simulink model "Project0x2DMPPTControl (2)"  (R2024a)
settings: Solver=FixedStepDiscrete  StartTime=0.0  StopTime=inf  FixedStep=10e-6  RelTol=1e-3
undefined symbols (not defined in the file): Ion, Lithium
libraries: spsSeriesRLCBranchLib x9, spsIGBTDiodeLib x3, slpidlib x2, spsPWMGeneratorDCDCLib x2, spsBatteryLib x1, spsCurrentMeasurementLib x1, spsDiodeLib x1, spsPVArrayLib x1, spsVoltageMeasurementLib x1, spspowerguiLib x1
settings Model: Creator=SHADMAN  LastModifiedBy=deept

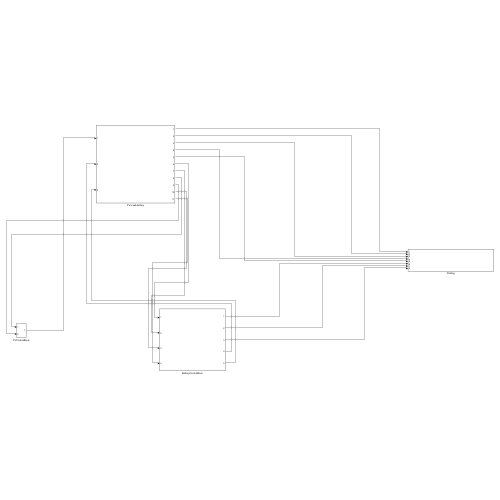
[thumbnail: Simulink's stored preview of the top-level diagram]
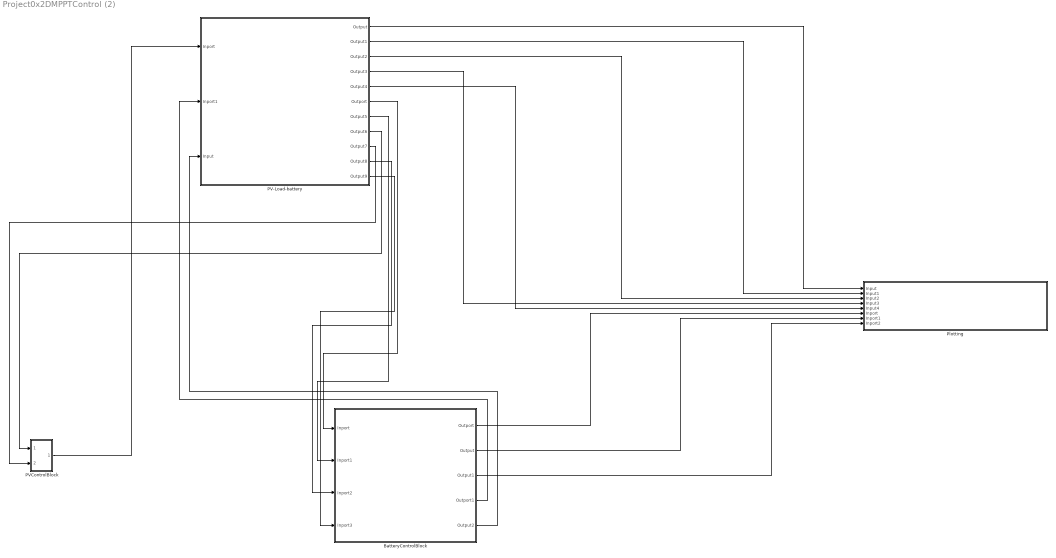
== system Project0x2DMPPTControl (2) ==
  BatteryControlBlock : Subsystem
  PV-Load-battery : Subsystem
  PVControlBlock : Subsystem
  Plotting : Subsystem
  wires:
  PV-Load-battery/1(Output) -> Plotting/1(Input)
  PV-Load-battery/2(Output1) -> Plotting/2(Input1)
  PV-Load-battery/4(Output3) -> Plotting/4(Input3)
  PV-Load-battery/5(Output4) -> Plotting/5(Input4)
  PV-Load-battery/3(Output2) -> Plotting/3(Input2)
  BatteryControlBlock/1(Outport) -> Plotting/6(Inport)
  BatteryControlBlock/2(Output) -> Plotting/7(Inport1)
  BatteryControlBlock/3(Output1) -> Plotting/8(Inport2)
  PVControlBlock/1(Outport) -> PV-Load-battery/1(Inport)
  PV-Load-battery/6(Outport) -> BatteryControlBlock/1(Inport)
  PV-Load-battery/7(Output5) -> BatteryControlBlock/2(Inport1)
  PV-Load-battery/8(Output6) -> PVControlBlock/1(Inport)
  PV-Load-battery/9(Output7) -> PVControlBlock/2(Input)
  PV-Load-battery/10(Output8) -> BatteryControlBlock/3(Inport2)
  PV-Load-battery/11(Output9) -> BatteryControlBlock/4(Inport3)
  BatteryControlBlock/4(Outport1) -> PV-Load-battery/2(Inport1)
  BatteryControlBlock/5(Output2) -> PV-Load-battery/3(Input)

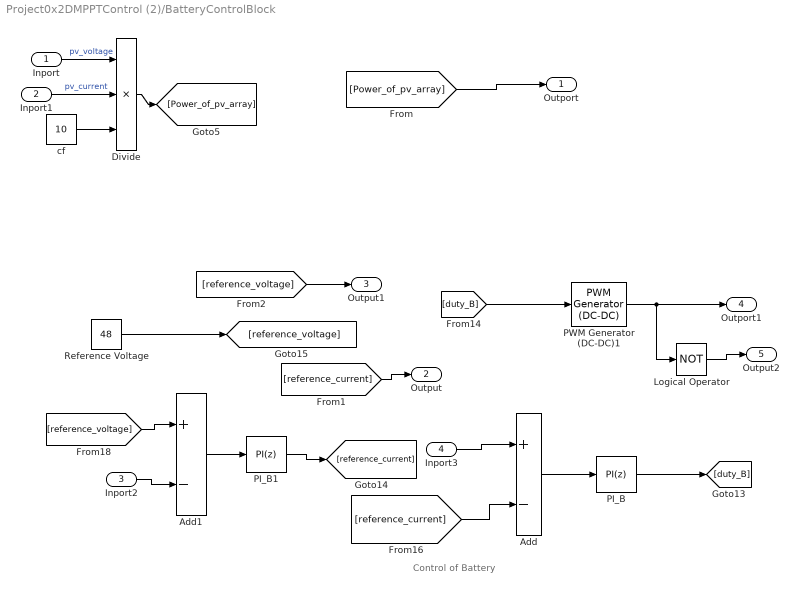
== system Project0x2DMPPTControl (2)/BatteryControlBlock ==
  note: Control of Battery
  Inport : Inport
  Inport1 : Inport  Port=2
  Inport2 : Inport  Port=3
  Inport3 : Inport  Port=4
  Add : Sum  Inputs=+-
  Add1 : Sum  Inputs=+-
  Divide : Product  Inputs=***
  Logical Operator : Logic  Operator=NOT  AllPortsSameDT=off  OutDataTypeStr=boolean
  PI_B : slpidlib/PID Controller  Controller=PI  Form=Parallel  TimeDomain=Discrete-time  UseExternalTs=off  SampleTime=50e-6  IntegratorMethod=Forward Euler  FilterMethod=Forward Euler  ControllerParametersSource=internal  P=0.01  I=10  UseKiTs=off  D=0  UseExternalDerivativeSource=off  N=100  UseFilter=on  TunerSelectOption=Transfer Function Based (PID Tuner App)  InitialConditionSource=internal  InitialConditionForIntegrator=0  InitialConditionForFilter=0  DifferentiatorICPrevScaledInput=0  ExternalReset=none  TrackingMode=off  Kt=1  LimitOutput=on  SatLimitsSource=internal  UpperSaturationLimit=0.95  LowerSaturationLimit=0  LinearizeAsGain=off  AntiWindupMode=none  Kb=1  LimitIntegrator=off  UpperIntegratorSaturationLimit=inf  LowerIntegratorSaturationLimit=-inf  POutMin=[]  POutMax=[]  IOutMin=[]  IOutMax=[]  DOutMin=[]  DOutMax=[]  NOutMin=[]  NOutMax=[]  SumOutMin=[]  SumOutMax=[]  SaturationOutMin=[]  SaturationOutMax=[]  PParamMin=[]  PParamMax=[]  IParamMin=[]  IParamMax=[]  DParamMin=[]  DParamMax=[]  NParamMin=[]  NParamMax=[]  KbParamMin=[]  KbParamMax=[]  KtParamMin=[]  KtParamMax=[]  KbOutMin=[]  KbOutMax=[]  KtOutMin=[]  KtOutMax=[]  IntegratorOutMin=[]  IntegratorOutMax=[]  FilterOutMin=[]  FilterOutMax=[]  SumI1OutMin=[]  SumI1OutMax=[]  SumI2OutMin=[]  SumI2OutMax=[]  SumI3OutMin=[]  SumI3OutMax=[]  SumI4OutMin=[]  SumI4OutMax=[]  SumDOutMin=[]  SumDOutMax=[]  DifferentiatorOutMin=[]  DifferentiatorOutMax=[]  FilterDiffOutCoefMin=[]  FilterDiffOutCoefMax=[]  ReciprocalOutMin=[]  ReciprocalOutMax=[]  SumDenOutMin=[]  SumDenOutMax=[]  SumNumOutMin=[]  SumNumOutMax=[]  DivideOutMin=[]  DivideOutMax=[]  UdiffTsProdOutMin=[]  UdiffTsProdOutMax=[]  NTsProdOutMin=[]  NTsProdOutMax=[]  UintegralTsProdOutMin=[]  UintegralTsProdOutMax=[]  UngainTsProdOutMin=[]  UngainTsProdOutMax=[]  ClampingZeroOutDataTypeStr=Inherit: Inherit via back propagation  ClampingZeroOutMin=[]  ClampingZeroOutMax=[]  FilterDenConstantOutDataTypeStr=Inherit: Inherit via back propagation  FilterDenConstantOutMin=[]  FilterDenConstantOutMax=[]  PCopyOutDataTypeStr=Inherit: Inherit via back propagation  PCopyOutMin=[]  PCopyOutMax=[]  NCopyOutDataTypeStr=Inherit: Inherit via back propagation  NCopyOutMin=[]  NCopyOutMax=[]  IntegratorContinuousStateAttributes=''  IntegratorStateMustResolveToSignalObject=off  IntegratorRTWStateStorageClass=Auto  FilterContinuousStateAttributes=''  FilterStateMustResolveToSignalObject=off  FilterRTWStateStorageClass=Auto  ParallelPVariant=InternalParameters  IdealPVariant=Disabled  IVariant=InternalParameters  DVariant=Disabled  IntegratorVariant=Discrete  SatVariant=Enabled  AWVariant=Passthrough  PCopyVariant=Disabled  TRVariant=Disabled  FdbkBlocksVariant=Forward  IdealPFdbkVariant=Disabled  SatFdbkVariant=Disabled  DerivativeFilterVariant=Disabled  NVariant=Disabled  NCopyVariant=Disabled_SignalSpec  FilterICVariant=Disabled  IntegratorICVariant=InternalICs  ExternalResetVariant=Disabled  TRSumVariant=Passthrough  SumFdbkVariant=Disabled  SumVariant=Sum_PI  TsampFilterVariant=InternalTs  TsampNgainVariant=Passthrough  TsampIntegralVariant=Disabled_SignalSpec  ExternalSaturationOutDataTypeStr=Inherit: Same as second input  DerivativeSourceVariant=Disabled
      settings: LibrarySourceBlock=simulink/Discrete/Discrete PID Controller
  PI_B1 : slpidlib/PID Controller  Controller=PI  Form=Parallel  TimeDomain=Discrete-time  UseExternalTs=off  SampleTime=500e-6  IntegratorMethod=Forward Euler  FilterMethod=Forward Euler  ControllerParametersSource=internal  P=0.85  I=10  UseKiTs=off  D=0  UseExternalDerivativeSource=off  N=100  UseFilter=on  TunerSelectOption=Transfer Function Based (PID Tuner App)  InitialConditionSource=internal  InitialConditionForIntegrator=0  InitialConditionForFilter=0  DifferentiatorICPrevScaledInput=0  ExternalReset=none  TrackingMode=off  Kt=1  LimitOutput=on  SatLimitsSource=internal  UpperSaturationLimit=22  LowerSaturationLimit=-22  LinearizeAsGain=off  AntiWindupMode=none  Kb=1  LimitIntegrator=off  UpperIntegratorSaturationLimit=inf  LowerIntegratorSaturationLimit=-inf  POutMin=[]  POutMax=[]  IOutMin=[]  IOutMax=[]  DOutMin=[]  DOutMax=[]  NOutMin=[]  NOutMax=[]  SumOutMin=[]  SumOutMax=[]  SaturationOutMin=[]  SaturationOutMax=[]  PParamMin=[]  PParamMax=[]  IParamMin=[]  IParamMax=[]  DParamMin=[]  DParamMax=[]  NParamMin=[]  NParamMax=[]  KbParamMin=[]  KbParamMax=[]  KtParamMin=[]  KtParamMax=[]  KbOutMin=[]  KbOutMax=[]  KtOutMin=[]  KtOutMax=[]  IntegratorOutMin=[]  IntegratorOutMax=[]  FilterOutMin=[]  FilterOutMax=[]  SumI1OutMin=[]  SumI1OutMax=[]  SumI2OutMin=[]  SumI2OutMax=[]  SumI3OutMin=[]  SumI3OutMax=[]  SumI4OutMin=[]  SumI4OutMax=[]  SumDOutMin=[]  SumDOutMax=[]  DifferentiatorOutMin=[]  DifferentiatorOutMax=[]  FilterDiffOutCoefMin=[]  FilterDiffOutCoefMax=[]  ReciprocalOutMin=[]  ReciprocalOutMax=[]  SumDenOutMin=[]  SumDenOutMax=[]  SumNumOutMin=[]  SumNumOutMax=[]  DivideOutMin=[]  DivideOutMax=[]  UdiffTsProdOutMin=[]  UdiffTsProdOutMax=[]  NTsProdOutMin=[]  NTsProdOutMax=[]  UintegralTsProdOutMin=[]  UintegralTsProdOutMax=[]  UngainTsProdOutMin=[]  UngainTsProdOutMax=[]  ClampingZeroOutDataTypeStr=Inherit: Inherit via back propagation  ClampingZeroOutMin=[]  ClampingZeroOutMax=[]  FilterDenConstantOutDataTypeStr=Inherit: Inherit via back propagation  FilterDenConstantOutMin=[]  FilterDenConstantOutMax=[]  PCopyOutDataTypeStr=Inherit: Inherit via back propagation  PCopyOutMin=[]  PCopyOutMax=[]  NCopyOutDataTypeStr=Inherit: Inherit via back propagation  NCopyOutMin=[]  NCopyOutMax=[]  IntegratorContinuousStateAttributes=''  IntegratorStateMustResolveToSignalObject=off  IntegratorRTWStateStorageClass=Auto  FilterContinuousStateAttributes=''  FilterStateMustResolveToSignalObject=off  FilterRTWStateStorageClass=Auto  ParallelPVariant=InternalParameters  IdealPVariant=Disabled  IVariant=InternalParameters  DVariant=Disabled  IntegratorVariant=Discrete  SatVariant=Enabled  AWVariant=Passthrough  PCopyVariant=Disabled  TRVariant=Disabled  FdbkBlocksVariant=Forward  IdealPFdbkVariant=Disabled  SatFdbkVariant=Disabled  DerivativeFilterVariant=Disabled  NVariant=Disabled  NCopyVariant=Disabled_SignalSpec  FilterICVariant=Disabled  IntegratorICVariant=InternalICs  ExternalResetVariant=Disabled  TRSumVariant=Passthrough  SumFdbkVariant=Disabled  SumVariant=Sum_PI  TsampFilterVariant=InternalTs  TsampNgainVariant=Passthrough  TsampIntegralVariant=Disabled_SignalSpec  ExternalSaturationOutDataTypeStr=Inherit: Same as second input  DerivativeSourceVariant=Disabled
      settings: LibrarySourceBlock=simulink/Discrete/Discrete PID Controller
  PWM Generator (DC-DC)1 : spsPWMGeneratorDCDCLib/PWM Generator (DC-DC)  Fsw=5000  Ts=10e-6
  Reference Voltage : Constant  Value=48
  cf : Constant  Value=10
  Outport : Outport
  Output : Outport  Port=2
  Output1 : Outport  Port=3
  Outport1 : Outport  Port=4
  Output2 : Outport  Port=5
  wires:
  Inport1/1 -> Divide/2  "pv_current"
  Divide/1 -> [Power_of_pv_array]
  Add/1 -> PI_B/1
  [duty_B] -> PWM Generator (DC-DC)1/1
  PWM Generator (DC-DC)1/1 -> Outport1/1, Logical Operator/1
  [reference_voltage] -> Add1/1
  [reference_current] -> Add/2
  Add1/1 -> PI_B1/1
  PI_B1/1 -> [reference_current]
  PI_B/1 -> [duty_B]
  Reference Voltage/1 -> [reference_voltage]
  cf/1 -> Divide/3
  Inport/1 -> Divide/1  "pv_voltage"
  [Power_of_pv_array] -> Outport/1
  [reference_current] -> Output/1
  [reference_voltage] -> Output1/1
  Inport2/1 -> Add1/2
  Inport3/1 -> Add/1
  Logical Operator/1 -> Output2/1

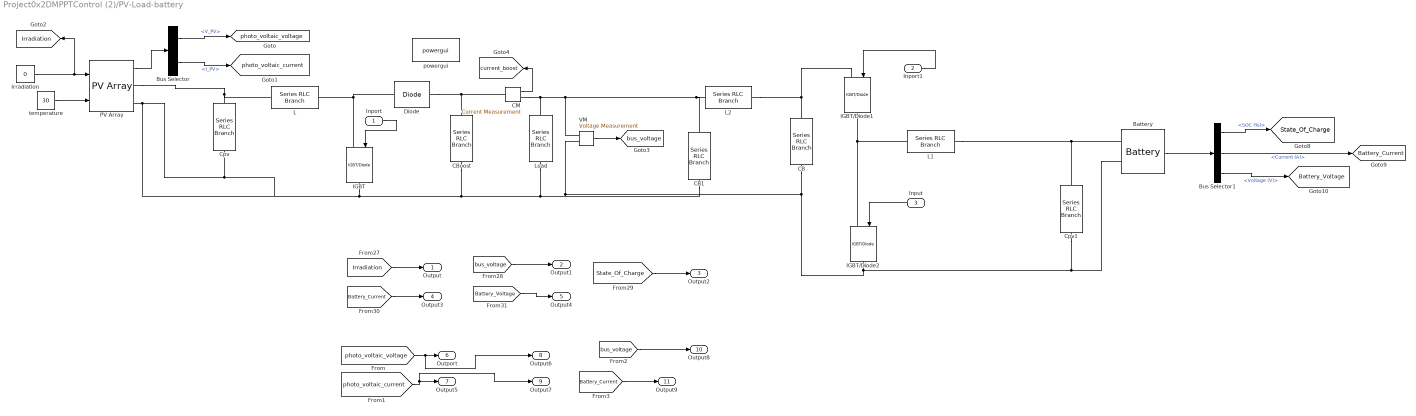
== system Project0x2DMPPTControl (2)/PV-Load-battery ==
  Inport : Inport
  Inport1 : Inport  Port=2
  Input : Inport  Port=3
  Battery : spsBatteryLib/Battery  BatType=Lithium-Ion  ShowTempParam=off  ThermalPreset=no  ShowAgeParam=off  NomV=24  NomQ=50  SOC=45  Batt_Tr=1  PresetModel=on  MaxQ=50  MinV=18  FullV=27.9357  Dis_rate=21.7391  R=0.0048  Normal_OP=45.2174  expZone="[25.9293      2.45652]"  current=[6.5 13 32.5]  Units=Time  Tci=20  NomT=20  T2=-30  MaxQ2=4.8  FullV2=7.1  Normal_OP2=5.655  expZone2="[6.58           1]"  Rca=0.6  ti=2000  Dp=0  Neq0=0  Tsim=1e6  Ta1=25  Qeol=5.4*0.9  Reol=0.013333*1.2  Char_age=[2.3478, 3]  Dis_age=[2.3478, 10]  N1=1500  N2=10500  N3=1000  N4=1400  Ta2=45  N5=950
  Bus Selector : BusSelector  OutputSignals=V_PV,I_PV
  Bus Selector1 : BusSelector  OutputSignals=SOC (%),Current (A),Voltage (V)
  CB : spsSeriesRLCBranchLib/Series RLC Branch  LConnTagsString=__new0  RConnTagsString=__new0  BranchType=RC  Resistance=1e-4  Inductance=1e-3  SetiL0=off  InitialCurrent=0  Capacitance=1000e-6  Setx0=off  InitialVoltage=0  Measurements=None
  CB1 : spsSeriesRLCBranchLib/Series RLC Branch  LConnTagsString=__new0  RConnTagsString=__new0  BranchType=RC  Resistance=1e-4  Inductance=1e-3  SetiL0=off  InitialCurrent=0  Capacitance=1000e-6  Setx0=off  InitialVoltage=0  Measurements=None
  CBoost : spsSeriesRLCBranchLib/Series RLC Branch  LConnTagsString=__new0  RConnTagsString=__new0  BranchType=RC  Resistance=1e-4  Inductance=1e-3  SetiL0=off  InitialCurrent=0  Capacitance=3300e-6  Setx0=off  InitialVoltage=0  Measurements=None
  CM : spsCurrentMeasurementLib/Current Measurement  PhasorSimulation=off  OutputType=Complex  PSBequivalent=0
  Cpv : spsSeriesRLCBranchLib/Series RLC Branch  LConnTagsString=__new0  RConnTagsString=__new0  BranchType=RC  Resistance=1e-4  Inductance=1e-3  SetiL0=off  InitialCurrent=0  Capacitance=100e-6  Setx0=off  InitialVoltage=0  Measurements=None
  Cpv1 : spsSeriesRLCBranchLib/Series RLC Branch  LConnTagsString=__new0  RConnTagsString=__new0  BranchType=RC  Resistance=0  Inductance=1e-3  SetiL0=off  InitialCurrent=0  Capacitance=1e-9  Setx0=off  InitialVoltage=0  Measurements=None
  Diode : spsDiodeLib/Diode  Ron=0.001  Lon=0  Vf=0.8  IC=0  UseSnubber=0  Rs=500  Cs=250e-9  Measurements=off
  IGBT : spsIGBTDiodeLib/IGBT//Diode  Ron=1e-3  Rs=1e5  Cs=inf  Measurements=off
  IGBT/Diode1 : spsIGBTDiodeLib/IGBT//Diode  Ron=1e-3  Rs=1e5  Cs=inf  Measurements=off
  IGBT/Diode2 : spsIGBTDiodeLib/IGBT//Diode  Ron=1e-3  Rs=1e5  Cs=inf  Measurements=off
  Irradiation : Constant  Value=0
  L : spsSeriesRLCBranchLib/Series RLC Branch  LConnTagsString=__new0  RConnTagsString=__new0  BranchType=RL  Resistance=0.1  Inductance=5e-3  SetiL0=off  InitialCurrent=0  Capacitance=100e-6  Setx0=off  InitialVoltage=0  Measurements=None
  L1 : spsSeriesRLCBranchLib/Series RLC Branch  LConnTagsString=__new0  RConnTagsString=__new0  BranchType=RL  Resistance=0.1  Inductance=1e-3  SetiL0=off  InitialCurrent=0  Capacitance=100e-6  Setx0=off  InitialVoltage=0  Measurements=None
  L2 : spsSeriesRLCBranchLib/Series RLC Branch  LConnTagsString=__new0  RConnTagsString=__new0  BranchType=RL  Resistance=0.1  Inductance=0.5e-3  SetiL0=off  InitialCurrent=0  Capacitance=100e-6  Setx0=off  InitialVoltage=0  Measurements=None
  Load : spsSeriesRLCBranchLib/Series RLC Branch  LConnTagsString=__new0  RConnTagsString=__new0  BranchType=R  Resistance=6  Inductance=1e-3  SetiL0=off  InitialCurrent=0  Capacitance=3300e-6  Setx0=off  InitialVoltage=0  Measurements=None
  PV Array : spsPVArrayLib/PV Array  Npar=5  Nser=1  PlotType=array @ 1000 W/m2 & specified temperatures  S_vec="[ 1000  500  100 ]"  Temp_C_vec="[ 45 25  ]"  ModuleName=User-defined  PlotWhenSelected=off  Pm=213.15  Ncell=60  Voc=36.3  Isc=7.84  Vm=29  Im=7.35  beta_Voc_pc=-0.36099  alpha_Isc_pc=0.102  beta_Voc=-0.13104  alpha_Isc=0.0079968  IL=7.8654  I0=2.9273e-10  nI=0.98119  Rsh=313.0553  Rs=0.39381  RobustModel=off  RobustCellTemperature=313.3991  BAL=on  Tc=1e-6  Tfilter=5e-5
  VM : spsVoltageMeasurementLib/Voltage Measurement  PhasorSimulation=off  OutputType=Complex  PSBequivalent=0
  powergui : spspowerguiLib/powergui  Priority=1  SimulationMode=Discrete  SampleTime=10e-6  frequency=60  Iterations=50  frequencyindice=0  Pbase=100e6  ErrMax=1e-4  UnitsV=kV  UnitsW=MW  buscounter=0  FunctionMessages=off  echomessages=off  EnableUseOfTLC=off  CurrentSourceSwitches=off  DisableSnubberDevices=off  DisableRonSwitches=off  DisableVfSwitches=off  DisplayEquations=off  AutomaticDiscreteSolvers=off  SolverType=Tustin/Backward Euler (TBE)  Interpol=off  ExternalGateDelay=off  methode=off  Ts=100  x0status=blocks  SPID=on  SwTol=0  HookPort=off  NonlinearTolerance=1e-4  nMaxIteration=100  ContinueOnMaxIteration=off  RestoreLinks=warning  ResistiveCurrentMeasurement=off  Frange=[0:2:500]  Ylog=off  Xlog=on  ShowGrid=off  save=off  variable=ZData  structure=0  ZoomFFT=off  StartTime=0.0  cycles=1  DisplayStyle=1  fundamental=60  FreqAxis=off  MaxFrequency=1000  frequencyindicesteady=1  RmsSteady=1  display=off
  temperature : Constant  Value=30
  Output : Outport
  Output1 : Outport  Port=2
  Output2 : Outport  Port=3
  Output3 : Outport  Port=4
  Output4 : Outport  Port=5
  Outport : Outport  Port=6
  Output5 : Outport  Port=7
  Output6 : Outport  Port=8
  Output7 : Outport  Port=9
  Output8 : Outport  Port=10
  Output9 : Outport  Port=11
  tag scope: Battery_Current=global, Battery_Voltage=global, Irradiation=global, State_Of_Charge=global, bus_voltage=global, current_boost=global, photo_voltaic_current=global, photo_voltaic_voltage=global
  wires:
  [Battery_Current] -> Output3/1
  [Battery_Voltage] -> Output4/1
  Bus Selector/1 -> [photo_voltaic_voltage]  "<V_PV>"
  CM/1 -> [current_boost]
  Bus Selector1/1 -> [State_Of_Charge]  "<SOC (%)>"
  Irradiation/1 -> [Irradiation], PV Array/1
  [bus_voltage] -> Output1/1
  [State_Of_Charge] -> Output2/1
  [Irradiation] -> Output/1
  Bus Selector/2 -> [photo_voltaic_current]  "<I_PV>"
  temperature/1 -> PV Array/2
  PV Array/1 -> Bus Selector/1
  VM/1 -> [bus_voltage]
  Input/1 -> IGBT/Diode2/1
  Bus Selector1/3 -> [Battery_Voltage]  "<Voltage (V)>"
  Inport/1 -> IGBT/1
  [photo_voltaic_voltage] -> Output6/1, Outport/1
  [photo_voltaic_current] -> Output7/1, Output5/1
  [bus_voltage] -> Output8/1
  [Battery_Current] -> Output9/1
  Inport1/1 -> IGBT/Diode1/1
  Battery/1 -> Bus Selector1/1
  Bus Selector1/2 -> [Battery_Current]  "<Current (A)>"
  connections:
  PV Array/RConn2 -- CB1/RConn1 -- Cpv/RConn1 -- Cpv1/RConn1 -- Battery/LConn2 -- IGBT/Diode2/RConn1 -- CB/RConn1 -- VM/LConn2 -- Load/RConn1 -- CBoost/RConn1 -- IGBT/RConn1
  Diode/RConn1 -- CM/LConn1 -- CBoost/LConn1
  IGBT/LConn1 -- Diode/LConn1 -- L/RConn1
  IGBT/Diode2/LConn1 -- L1/LConn1 -- IGBT/Diode1/RConn1
  CB/LConn1 -- IGBT/Diode1/LConn1 -- L2/RConn1
  PV Array/RConn1 -- L/LConn1 -- Cpv/LConn1
  L1/RConn1 -- Cpv1/LConn1 -- Battery/LConn1
  CM/RConn1 -- CB1/LConn1 -- L2/LConn1 -- VM/LConn1 -- Load/LConn1

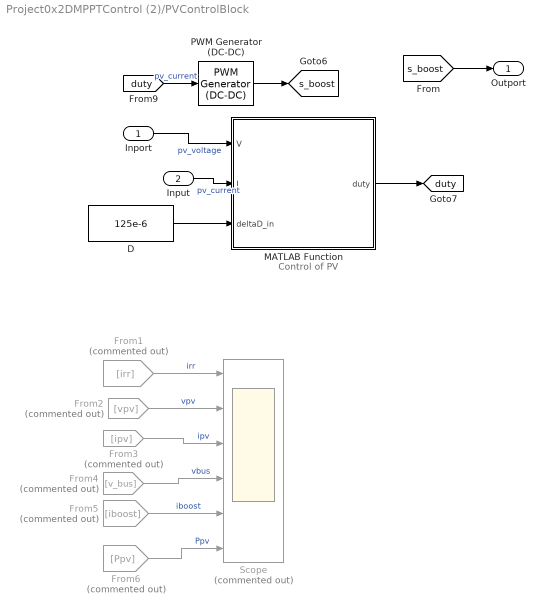
== system Project0x2DMPPTControl (2)/PVControlBlock ==
  note: Control of PV
  Inport : Inport
  Input : Inport  Port=2
  D : Constant  Value=125e-6
  From1 : From  Commented=on  GotoTag=irr  TagVisibility=global
  From2 : From  Commented=on  GotoTag=vpv  TagVisibility=global
  From3 : From  Commented=on  GotoTag=ipv  TagVisibility=global
  From4 : From  Commented=on  GotoTag=v_bus  TagVisibility=global
  From5 : From  Commented=on  GotoTag=iboost  TagVisibility=global
  From6 : From  Commented=on  GotoTag=Ppv
  MATLAB Function : MATLAB Function  TreatAsAtomicUnit=on
  PWM Generator (DC-DC) : spsPWMGeneratorDCDCLib/PWM Generator (DC-DC)  Fsw=5000  Ts=10e-6
  Scope : Scope  Commented=on  NumInputPorts=6
  Outport : Outport
  tag scope: duty=global, s_boost=global
  wires:
  D/1 -> MATLAB Function/3(deltaD_in)
  MATLAB Function/1(duty) -> [duty]
  PWM Generator (DC-DC)/1 -> [s_boost]
  [duty] -> PWM Generator (DC-DC)/1  "pv_current"
  From6/1 -> Scope/6  "Ppv"
  Input/1 -> MATLAB Function/2(I)  "pv_current"
  From2/1 -> Scope/2  "vpv"
  From4/1 -> Scope/4  "vbus"
  From1/1 -> Scope/1  "irr"
  From3/1 -> Scope/3  "ipv"
  From5/1 -> Scope/5  "iboost"
  Inport/1 -> MATLAB Function/1(V)  "pv_voltage"
  [s_boost] -> Outport/1

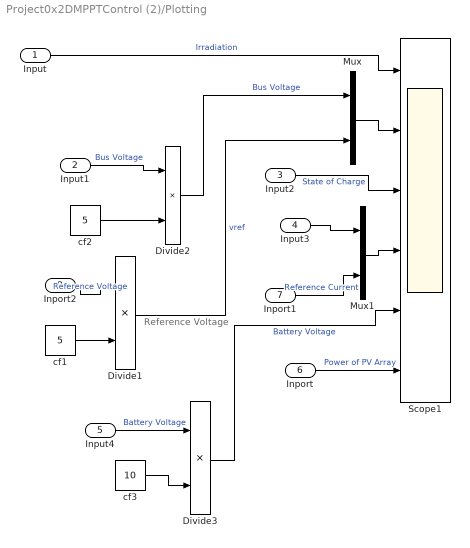
== system Project0x2DMPPTControl (2)/Plotting ==
  note: Reference Voltage
  Input : Inport
  Input1 : Inport  Port=2
  Input2 : Inport  Port=3
  Input3 : Inport  Port=4
  Input4 : Inport  Port=5
  Inport : Inport  Port=6
  Inport1 : Inport  Port=7
  Inport2 : Inport  Port=8
  Divide1 : Product  Inputs=**
  Divide2 : Product  Inputs=**
  Divide3 : Product  Inputs=**
  Mux : Mux  Inputs=2
  Mux1 : Mux  Inputs=2
  Scope1 : Scope  NumInputPorts=6
  cf1 : Constant  Value=5
  cf2 : Constant  Value=5
  cf3 : Constant  Value=10
  wires:
  cf1/1 -> Divide1/2
  Mux1/1 -> Scope1/4
  Inport1/1 -> Mux1/2  "Reference Current"
  Input/1 -> Scope1/1  "Irradiation"
  Input2/1 -> Scope1/3  "State of Charge"
  Divide1/1 -> Mux/2  "vref"
  Mux/1 -> Scope1/2
  Inport/1 -> Scope1/6  "Power of PV Array"
  Divide2/1 -> Mux/1  "Bus Voltage"
  cf3/1 -> Divide3/2
  cf2/1 -> Divide2/2
  Input1/1 -> Divide2/1  "Bus Voltage"
  Input4/1 -> Divide3/1  "Battery Voltage"
  Divide3/1 -> Scope1/5  "Battery Voltage"
  Inport2/1 -> Divide1/1  "Reference Voltage"
  Input3/1 -> Mux1/1

== matlab function Project0x2DMPPTControl (2)/PVControlBlock/MATLAB Function ==
  data: V input; duty output; I input; deltaD_in input
function duty = MPPT_Control( V, I,deltaD_in)

duty_init = 0.05;
duty_min=0;
duty_max=0.75;

persistent Vold Pold duty_old;

if isempty(Vold)
    Vold=0;
    Pold=0;
    duty_old=duty_init;
end
P= V*I;
dV= V - Vold;
dP= P - Pold;
duty = duty_old;
deltaD=deltaD_in;

if dP ~= 0
    if dP < 0
        if dV < 0
            duty = duty_old - deltaD;
        else
            duty = duty_old + deltaD;
        end
    else
        if dV < 0
            duty = duty_old + deltaD;
        else
            duty = duty_old - deltaD;
        end
    end
end

if duty >= duty_max
    duty=duty_max;
elseif duty<duty_min
    duty=duty_min;
end

duty_old=duty;
Vold=V;
Pold=P;
